simulink model "SensorMeasurements"  (R2023b)
settings: Solver=FixedStepAuto  StartTime=0.0  StopTime=10.0  FixedStep=0.001  RelTol=1e-3
settings Model: Creator=OWNER  LastModifiedBy=OWNER

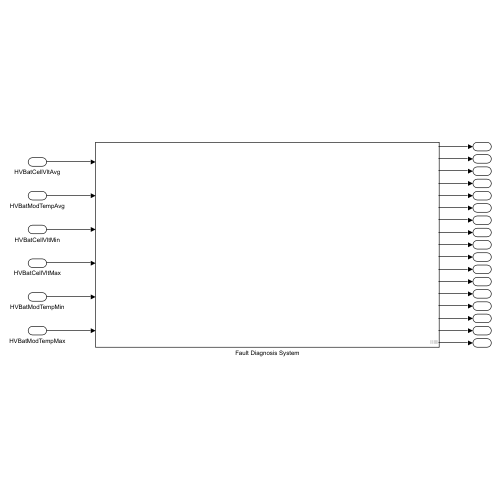
[thumbnail: Simulink's stored preview of the top-level diagram]
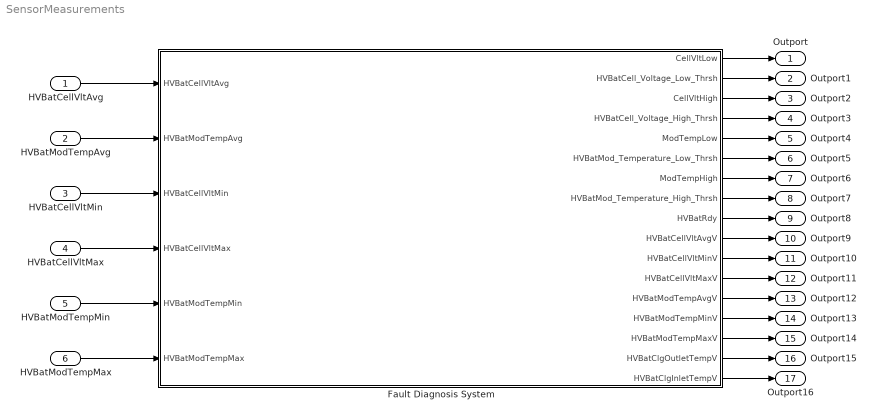
== system SensorMeasurements ==
  HVBatCellVltAvg : Inport
  HVBatModTempAvg : Inport  Port=2
  HVBatCellVltMin : Inport  Port=3
  HVBatCellVltMax : Inport  Port=4
  HVBatModTempMin : Inport  Port=5
  HVBatModTempMax : Inport  Port=6
  Fault Diagnosis System : Subsystem
  Outport : Outport
  Outport1 : Outport  Port=2
  Outport2 : Outport  Port=3
  Outport3 : Outport  Port=4
  Outport4 : Outport  Port=5
  Outport5 : Outport  Port=6
  Outport6 : Outport  Port=7
  Outport7 : Outport  Port=8
  Outport8 : Outport  Port=9
  Outport9 : Outport  Port=10
  Outport10 : Outport  Port=11
  Outport11 : Outport  Port=12
  Outport12 : Outport  Port=13
  Outport13 : Outport  Port=14
  Outport14 : Outport  Port=15
  Outport15 : Outport  Port=16
  Outport16 : Outport  Port=17
  wires:
  HVBatCellVltMin/1 -> Fault Diagnosis System/3(HVBatCellVltMin)
  HVBatCellVltMax/1 -> Fault Diagnosis System/4(HVBatCellVltMax)
  HVBatModTempMin/1 -> Fault Diagnosis System/5(HVBatModTempMin)
  HVBatModTempMax/1 -> Fault Diagnosis System/6(HVBatModTempMax)
  HVBatCellVltAvg/1 -> Fault Diagnosis System/1(HVBatCellVltAvg)
  HVBatModTempAvg/1 -> Fault Diagnosis System/2(HVBatModTempAvg)
  Fault Diagnosis System/1(CellVltLow) -> Outport/1
  Fault Diagnosis System/2(HVBatCell_Voltage_Low_Thrsh) -> Outport1/1
  Fault Diagnosis System/3(CellVltHigh) -> Outport2/1
  Fault Diagnosis System/4(HVBatCell_Voltage_High_Thrsh) -> Outport3/1
  Fault Diagnosis System/7(ModTempHigh) -> Outport6/1
  Fault Diagnosis System/8(HVBatMod_Temperature_High_Thrsh) -> Outport7/1
  Fault Diagnosis System/5(ModTempLow) -> Outport4/1
  Fault Diagnosis System/6(HVBatMod_Temperature_Low_Thrsh) -> Outport5/1
  Fault Diagnosis System/15(HVBatModTempMaxV) -> Outport14/1
  Fault Diagnosis System/16(HVBatClgOutletTempV) -> Outport15/1
  Fault Diagnosis System/14(HVBatModTempMinV) -> Outport13/1
  Fault Diagnosis System/13(HVBatModTempAvgV) -> Outport12/1
  Fault Diagnosis System/11(HVBatCellVltMinV) -> Outport10/1
  Fault Diagnosis System/12(HVBatCellVltMaxV) -> Outport11/1
  Fault Diagnosis System/9(HVBatRdy) -> Outport8/1
  Fault Diagnosis System/10(HVBatCellVltAvgV) -> Outport9/1
  Fault Diagnosis System/17(HVBatClgInletTempV) -> Outport16/1

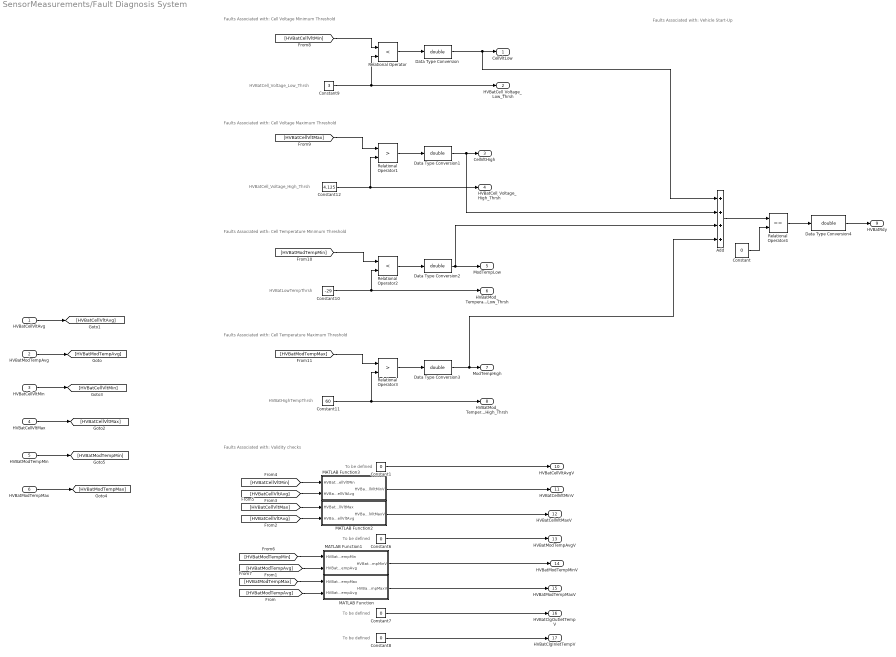
== system SensorMeasurements/Fault Diagnosis System ==
  note: Faults Associated with: Validity checks
  note: Faults Associated with: Vehicle Start-Up
  note: Faults Associated with: Cell Temperature Minimum Threshold
  note: Faults Associated with: Cell Voltage Maximum Threshold
  note: Faults Associated with: Cell Voltage Minimum Threshold
  note: Faults Associated with: Cell Temperature Maximum Threshold
  note: To be defined
  note: To be defined
  note: To be defined
  note: To be defined
  note: HVBatLowTempThrsh
  note: HVBatHighTempThrsh
  note: HVBatCell_Voltage_Low_Thrsh
  note: HVBatCell_Voltage_High_Thrsh
  HVBatCellVltAvg : Inport
  HVBatModTempAvg : Inport  Port=2
  HVBatCellVltMin : Inport  Port=3
  HVBatCellVltMax : Inport  Port=4
  HVBatModTempMin : Inport  Port=5
  HVBatModTempMax : Inport  Port=6
  Add : Sum  Inputs=++++
  Constant{,1,6..8} (5 alike) : Constant  Value=0
  Constant10 : Constant  Value=-29
  Constant11 : Constant  Value=60
  Constant12 : Constant  Value=4.125
  Constant9 : Constant  Value=3
  Data Type Conversion{,1..4} (5 alike) : DataTypeConversion  OutDataTypeStr=double  SaturateOnIntegerOverflow=off  RndMeth=Floor
  MATLAB Function : MATLAB Function  TreatAsAtomicUnit=on
  MATLAB Function1 : MATLAB Function  TreatAsAtomicUnit=on
  MATLAB Function2 : MATLAB Function  TreatAsAtomicUnit=on
  MATLAB Function3 : MATLAB Function  TreatAsAtomicUnit=on
  Relational Operator : RelationalOperator  Operator=<  OutDataTypeStr=boolean  RndMeth=Simplest  InputSameDT=off
  Relational Operator1 : RelationalOperator  Operator=>  OutDataTypeStr=boolean  RndMeth=Simplest  InputSameDT=off
  Relational Operator2 : RelationalOperator  Operator=<  OutDataTypeStr=boolean  RndMeth=Simplest  InputSameDT=off
  Relational Operator3 : RelationalOperator  Operator=>  OutDataTypeStr=boolean  RndMeth=Simplest  InputSameDT=off
  Relational Operator4 : RelationalOperator  Operator===  OutDataTypeStr=boolean  RndMeth=Simplest  InputSameDT=off
  CellVltLow : Outport
  HVBatCell_Voltage_Low_Thrsh : Outport  Port=2
  CellVltHigh : Outport  Port=3
  HVBatCell_Voltage_High_Thrsh : Outport  Port=4
  ModTempLow : Outport  Port=5
  HVBatMod_Temperature_Low_Thrsh : Outport  Port=6
  ModTempHigh : Outport  Port=7
  HVBatMod_Temperature_High_Thrsh : Outport  Port=8
  HVBatRdy : Outport  Port=9
  HVBatCellVltAvgV : Outport  Port=10
  HVBatCellVltMinV : Outport  Port=11
  HVBatCellVltMaxV : Outport  Port=12
  HVBatModTempAvgV : Outport  Port=13
  HVBatModTempMinV : Outport  Port=14
  HVBatModTempMaxV : Outport  Port=15
  HVBatClgOutletTempV : Outport  Port=16
  HVBatClgInletTempV : Outport  Port=17
  wires:
  [HVBatCellVltMin] -> Relational Operator/1
  Relational Operator/1 -> Data Type Conversion/1
  Data Type Conversion/1 -> CellVltLow/1, Add/1
  [HVBatCellVltMax] -> Relational Operator1/1
  Relational Operator1/1 -> Data Type Conversion1/1
  Data Type Conversion1/1 -> CellVltHigh/1, Add/2
  Data Type Conversion2/1 -> Add/3, ModTempLow/1
  Constant10/1 -> HVBatMod_Temperature_Low_Thrsh/1, Relational Operator2/2
  Relational Operator2/1 -> Data Type Conversion2/1
  [HVBatModTempMin] -> Relational Operator2/1
  Data Type Conversion3/1 -> ModTempHigh/1, Add/4
  Relational Operator3/1 -> Data Type Conversion3/1
  [HVBatModTempMax] -> Relational Operator3/1
  Add/1 -> Relational Operator4/1
  Constant/1 -> Relational Operator4/2
  Relational Operator4/1 -> Data Type Conversion4/1
  MATLAB Function2/1(HVBatCellVltMaxV) -> HVBatCellVltMaxV/1
  MATLAB Function3/1(HVBatCellVltMinV) -> HVBatCellVltMinV/1
  Constant1/1 -> HVBatCellVltAvgV/1
  MATLAB Function/1(HVBatModTempMaxV) -> HVBatModTempMaxV/1
  Constant6/1 -> HVBatModTempAvgV/1
  MATLAB Function1/1(HVBatModTempMinV) -> HVBatModTempMinV/1
  Constant7/1 -> HVBatClgOutletTempV/1
  Constant8/1 -> HVBatClgInletTempV/1
  Constant11/1 -> HVBatMod_Temperature_High_Thrsh/1, Relational Operator3/2
  Constant12/1 -> HVBatCell_Voltage_High_Thrsh/1, Relational Operator1/2
  Constant9/1 -> HVBatCell_Voltage_Low_Thrsh/1, Relational Operator/2
  Data Type Conversion4/1 -> HVBatRdy/1
  [HVBatModTempAvg] -> MATLAB Function/2(HVBatModTempAvg)
  [HVBatModTempAvg] -> MATLAB Function1/2(HVBatModTempAvg)
  HVBatCellVltAvg/1 -> [HVBatCellVltAvg]
  HVBatModTempAvg/1 -> [HVBatModTempAvg]
  HVBatCellVltMax/1 -> [HVBatCellVltMax]
  HVBatCellVltMin/1 -> [HVBatCellVltMin]
  HVBatModTempMax/1 -> [HVBatModTempMax]
  HVBatModTempMin/1 -> [HVBatModTempMin]
  [HVBatCellVltAvg] -> MATLAB Function2/2(HVBatCellVltAvg)
  [HVBatCellVltAvg] -> MATLAB Function3/2(HVBatCellVltAvg)
  [HVBatCellVltMin] -> MATLAB Function3/1(HVBatCellVltMin)
  [HVBatCellVltMax] -> MATLAB Function2/1(HVBatCellVltMax)
  [HVBatModTempMin] -> MATLAB Function1/1(HVBatModTempMin)
  [HVBatModTempMax] -> MATLAB Function/1(HVBatModTempMax)

== matlab function SensorMeasurements/Fault Diagnosis System/MATLAB Function1 ==
  data: HVBatModTempMin input; HVBatModTempMinV output; HVBatModTempAvg input
function HVBatModTempMinV = checkTempMinValidity(HVBatModTempMin, HVBatModTempAvg)

% Constants
TEMP_THRESHOLD = 10;   % degC
TIME_WINDOW_MS = 100;  % 100 ms
TS_MS          = 1;    % fixed step = 1 ms

VALID     = 0;
NOT_VALID = 1;

% Persistent counter (ms)
persistent violationTimeMs

if isempty(violationTimeMs)
    violationTimeMs = 0;
end

% Deviation from average
devMin = abs(HVBatModTempMin - HVBatModTempAvg);

% Threshold check
if devMin > TEMP_THRESHOLD
    violationTimeMs = violationTimeMs + TS_MS;
else
    violationTimeMs = 0;
end

% Validity decision
if violationTimeMs >= TIME_WINDOW_MS
    HVBatModTempMinV = NOT_VALID;
else
    HVBatModTempMinV = VALID;
end

== matlab function SensorMeasurements/Fault Diagnosis System/MATLAB Function2 ==
  data: HVBatCellVltMax input; HVBatCellVltMaxV output; HVBatCellVltAvg input
function HVBatCellVltMaxV = checkVltMaxValidity(HVBatCellVltMax, HVBatCellVltAvg)

% Constants
VLT_THRESHOLD = 1.7;     % Volts
TIME_WINDOW_MS = 100; % 100 ms
TS_MS          = 1;   % fixed step = 1 ms

VALID     = 0;
NOT_VALID = 1;

% Persistent counter (ms)
persistent violationTimeMs

if isempty(violationTimeMs)
    violationTimeMs = 0;
end

% Deviation from average
devMax = abs(HVBatCellVltMax - HVBatCellVltAvg);

% Threshold check
if devMax > VLT_THRESHOLD
    violationTimeMs = violationTimeMs + TS_MS;
else
    violationTimeMs = 0;
end

% Validity decision
if violationTimeMs >= TIME_WINDOW_MS
    HVBatCellVltMaxV = NOT_VALID;
else
    HVBatCellVltMaxV = VALID;
end

== matlab function SensorMeasurements/Fault Diagnosis System/MATLAB Function3 ==
  data: HVBatCellVltMin input; HVBatCellVltMinV output; HVBatCellVltAvg input
function HVBatCellVltMinV = checkVltMinValidity(HVBatCellVltMin, HVBatCellVltAvg)

% Constants
VLT_THRESHOLD = 1.7;     % Volts
TIME_WINDOW_MS = 100; % 100 ms
TS_MS          = 1;   % fixed step = 1 ms

VALID     = 0;
NOT_VALID = 1;

% Persistent counter (ms)
persistent violationTimeMs

if isempty(violationTimeMs)
    violationTimeMs = 0;
end

% Deviation from average
devMin = abs(HVBatCellVltMin - HVBatCellVltAvg);

% Threshold check
if devMin > VLT_THRESHOLD
    violationTimeMs = violationTimeMs + TS_MS;
else
    violationTimeMs = 0;
end

% Validity decision
if violationTimeMs >= TIME_WINDOW_MS
    HVBatCellVltMinV = NOT_VALID;
else
    HVBatCellVltMinV = VALID;
end

== matlab function SensorMeasurements/Fault Diagnosis System/MATLAB Function ==
  data: HVBatModTempMax input; HVBatModTempMaxV output; HVBatModTempAvg input
function HVBatModTempMaxV = checkTempMaxValidity(HVBatModTempMax, HVBatModTempAvg)

% Constants
TEMP_THRESHOLD = 10;   % degC
TIME_WINDOW_MS = 100;  % 100 ms
TS_MS          = 1;    % fixed step = 1 ms

VALID     = 0;
NOT_VALID = 1;

% Persistent counter (ms)
persistent violationTimeMs

if isempty(violationTimeMs)
    violationTimeMs = 0;
end

% Deviation from average
devMax = abs(HVBatModTempMax - HVBatModTempAvg);

% Threshold check
if devMax > TEMP_THRESHOLD
    violationTimeMs = violationTimeMs + TS_MS;
else
    violationTimeMs = 0;
end

% Validity decision
if violationTimeMs >= TIME_WINDOW_MS
    HVBatModTempMaxV = NOT_VALID;
else
    HVBatModTempMaxV = VALID;
end
